simulink model "unit_membrane"  (R2025a)
settings: Solver=VariableStepAuto  StartTime=0.0  StopTime=1000000  RelTol=1e-3
libraries: nesl_utility x1
settings Model: Creator=degoede  LastModifiedBy=degoede
settings SimscapeCC: SimscapeLogType=all  SimscapeLogOpenViewer=on

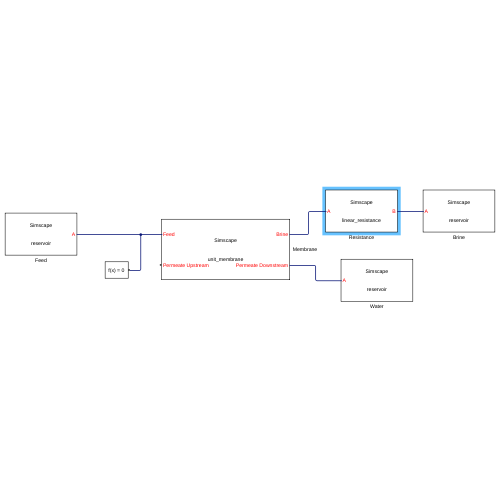
[thumbnail: Simulink's stored preview of the top-level diagram]
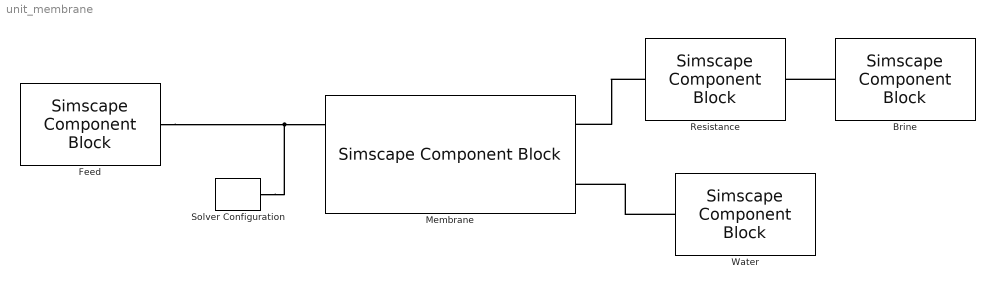
== system unit_membrane ==
  Brine : SimscapeComponentBlock  SourceFile=customization.solution.elements.reservoir  ComponentPath=customization.solution.elements.reservoir  ComponentVariants="[\"customization.solution.elements.reservoir\"]"  ComponentVariantNames="[\"reservoir\"]"  ClassName=reservoir  SchemaVersion=1  pressure_spec=foundation.enum.pressure_spec.atmospheric  reservoir_pressure=0.101325 MPa  reservoir_temperature=293.15 K  reservoir_concentration=50 kg/m^3  area=27 mm^2
      settings: CopyFcn=simscape.sscblock.internal.componentBlockCallback(gcbh,'COPY')  PreCopyFcn=simscape.sscblock.internal.componentBlockCallback(gcbh,'PRECOPY')  PreDeleteFcn=simscape.sscblock.internal.componentBlockCallback(gcbh,'PREDELETE')  InternalSimscapePortConfiguration="{\"Bottom\":[],\"Left\":[{\"id\":\"A\",\"label\":\"A\",\"type\":\"customization.solution.solution\"}],\"Right\":[],\"Top\":[]}"
      mask Type: Reservoir (SS)
  Feed : SimscapeComponentBlock  SourceFile=customization.solution.elements.reservoir  ComponentPath=customization.solution.elements.reservoir  ComponentVariants="[\"customization.solution.elements.reservoir\"]"  ComponentVariantNames="[\"reservoir\"]"  ClassName=reservoir  SchemaVersion=1  pressure_spec=foundation.enum.pressure_spec.specified  reservoir_pressure=5 MPa  reservoir_temperature=293.15 K  reservoir_concentration=32 kg/m^3  area=1 cm^2
      settings: CopyFcn=simscape.sscblock.internal.componentBlockCallback(gcbh,'COPY')  PreCopyFcn=simscape.sscblock.internal.componentBlockCallback(gcbh,'PRECOPY')  PreDeleteFcn=simscape.sscblock.internal.componentBlockCallback(gcbh,'PREDELETE')  InternalSimscapePortConfiguration="{\"Bottom\":[],\"Left\":[{\"id\":\"A\",\"label\":\"A\",\"type\":\"customization.solution.solution\"}],\"Right\":[],\"Top\":[]}"
      mask Type: Reservoir (SS)
  Membrane : SimscapeComponentBlock  SourceFile=customization.solution.elements.unit_membrane  ComponentPath=customization.solution.elements.unit_membrane  ComponentVariants="[\"customization.solution.elements.unit_membrane\"]"  ComponentVariantNames="[\"unit_membrane\"]"  ClassName=unit_membrane  SchemaVersion=1  A_w=2.57e-12 m^3/(N*s)  B_s=2.30e-8 m/s  A_m=35 m^2  length=1 m  D_feed=0.7556 mm  area_feed=604.5200 mm^2  D_perm=29 mm  P0_feed=5 MPa  P0_perm=0.101 MPa  x0_feed=32 kg/m^3  x0_perm=0 kg/m^3  roughness=15e-6 m  Re_lam=2000  Re_tur=4000  shape_factor=64  Nu_lam=3.66
      settings: CopyFcn=simscape.sscblock.internal.componentBlockCallback(gcbh,'COPY')  PreCopyFcn=simscape.sscblock.internal.componentBlockCallback(gcbh,'PRECOPY')  PreDeleteFcn=simscape.sscblock.internal.componentBlockCallback(gcbh,'PREDELETE')  InternalSimscapePortConfiguration="{\"Bottom\":[],\"Left\":[{\"id\":\"F\",\"label\":\"Feed\",\"type\":\"customization.solution.solution\"},{\"id\":\"P1\",\"label\":\"Permeate Upstream\",\"type\":\"customization.solution.solution\"}],\"Right\":[{\"id\":\"B\",\"label\":\"Brine\",\"type\":\"customization.solution.solution\"},{\"id\":\"P2\",\"label\":\"Permeate Downstream\",\"type\":\"customization.solution.solution\"}],\"Top\":[]}"
      mask Type: Unit Membrane (SS)
  Resistance : SimscapeComponentBlock  SourceFile=customization.solution.elements.linear_resistance  ComponentPath=customization.solution.elements.linear_resistance  ComponentVariants="[\"customization.solution.elements.linear_resistance\"]"  ComponentVariantNames="[\"linear_resistance\"]"  ClassName=linear_resistance  SchemaVersion=1  R=64.23e8 Pa*s/m^3  area=0.01 m^2
      settings: CopyFcn=simscape.sscblock.internal.componentBlockCallback(gcbh,'COPY')  PreCopyFcn=simscape.sscblock.internal.componentBlockCallback(gcbh,'PRECOPY')  PreDeleteFcn=simscape.sscblock.internal.componentBlockCallback(gcbh,'PREDELETE')  InternalSimscapePortConfiguration="{\"Bottom\":[],\"Left\":[{\"id\":\"A\",\"label\":\"A\",\"type\":\"customization.solution.solution\"}],\"Right\":[{\"id\":\"B\",\"label\":\"B\",\"type\":\"customization.solution.solution\"}],\"Top\":[]}"
      mask Type: Linear Resistance (SS)
  Solver Configuration : nesl_utility/Solver Configuration  PhysicalDomain=network_engine_domain  SubClassName=solver  LeftPortType=input  RightPortType=generic  Tones=[]  Harmonics=[]  SimulateNoise=off  Profile=off  UseLocalSampling=off  EnableSwitchedLinearOptims=on  FrequencyDomain=off  UseCCode=off  RelTol=0.001  AbsTol=0.001  MinStep=1e-09  ToWorkspace=off  RevertToSquareIcSolve=off  NumHomotopyIterations=100  PhasorMode=off  PhasorModeNumHarmonics=1  ConsistencySolver=NEWTON_XTOL_AFTER_FTOL  IndexReductionMethod=DerivativeReplacement  DoDC=off  ResidualTolerance=1e-09  ConsistencyTolSource=GLOBAL  ConsistencyAbsTol=0.001  ConsistencyRelTol=0.001  ConsistencyTolFactor=0.001  UseLocalSolver=off  LocalSolverChoice=NE_BACKWARD_EULER_ADVANCER  ResolveIndetEquations=on  FunctionEvalNumThread=1  LocalSolverSampleTime=0.001  DoFixedCost=off  MaxNonlinIter=3  MaxModeIter=2  ComputeImpulses=off  ImpulseIterations=2  LinearAlgebra=auto  LinearAlgebraNumThread=0  EquationFormulation=NE_TIME_EF  DelaysMemoryBudget=1024  AutomaticFiltering=off  FilteringTimeConstant=0.001  PartitionStorageMethod=AS_NEEDED  PartitionMemoryBudget=1024  PartitionMethod=ROBUST  MultibodyUseLocalSolver=off  MultibodyLocalSolverChoice=ODE1  MultibodyLocalSolverSampleTime=0.001
  Water : SimscapeComponentBlock  SourceFile=customization.solution.elements.reservoir  ComponentPath=customization.solution.elements.reservoir  ComponentVariants="[\"customization.solution.elements.reservoir\"]"  ComponentVariantNames="[\"reservoir\"]"  ClassName=reservoir  SchemaVersion=1  pressure_spec=foundation.enum.pressure_spec.atmospheric  reservoir_pressure=0.101325 MPa  reservoir_temperature=293.15 K  reservoir_concentration=0 kg/m^3  area=1 cm^2
      settings: CopyFcn=simscape.sscblock.internal.componentBlockCallback(gcbh,'COPY')  PreCopyFcn=simscape.sscblock.internal.componentBlockCallback(gcbh,'PRECOPY')  PreDeleteFcn=simscape.sscblock.internal.componentBlockCallback(gcbh,'PREDELETE')  InternalSimscapePortConfiguration="{\"Bottom\":[],\"Left\":[{\"id\":\"A\",\"label\":\"A\",\"type\":\"customization.solution.solution\"}],\"Right\":[],\"Top\":[]}"
      mask Type: Reservoir (SS)
  connections:
  Solver Configuration/RConn1 -- Feed/LConn1 -- Membrane/LConn1
  Brine/LConn1 -- Resistance/RConn1
  Water/LConn1 -- Membrane/RConn2
  Resistance/LConn1 -- Membrane/RConn1
